simulink model "linear_observor"  (R2023a)
settings: Solver=VariableStepAuto  StartTime=0.0  StopTime=50  RelTol=1e-3
settings Model: Creator=belov  LastModifiedBy=belov

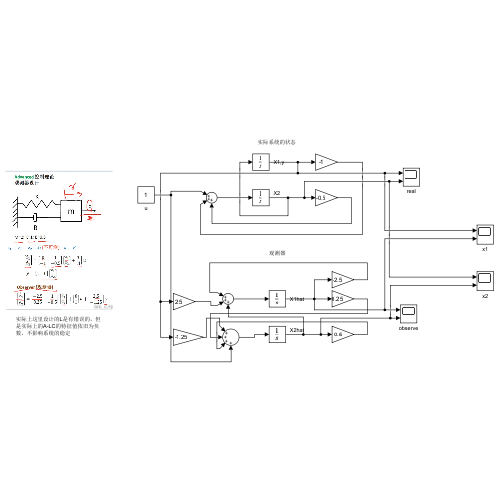
[thumbnail: Simulink's stored preview of the top-level diagram]
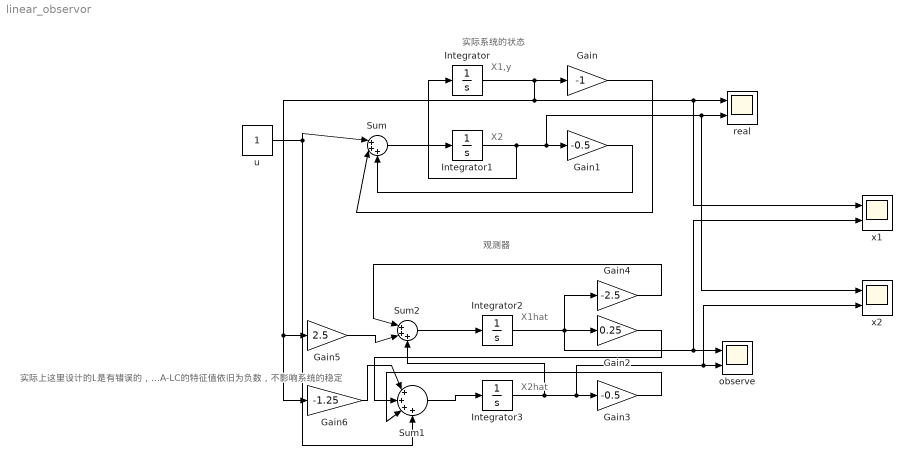
== system linear_observor ==
  note: 实际上这里设计的L是有错误的，但是实际上的A-LC的特征值依旧为负数，不影响系统的稳定
  note: 观测器
  note: 实际系统的状态
  note: X2
  note: X1,y
  note: X2hat
  note: X1hat
  Gain : Gain  Gain=-1
  Gain1 : Gain  Gain=-0.5
  Gain2 : Gain  Gain=0.25
  Gain3 : Gain  Gain=-0.5
  Gain4 : Gain  Gain=-2.5
  Gain5 : Gain  Gain=2.5
  Gain6 : Gain  Gain=-1.25
  Integrator{,1..3} (4 alike) : Integrator
  Sum : Sum  Inputs=|+++
  Sum1 : Sum  Inputs=|++++
  Sum2 : Sum  Inputs=|+++
  observe : Scope  NumInputPorts=2
  real : Scope  NumInputPorts=2
  u : Constant
  x1 : Scope  NumInputPorts=2
  x2 : Scope  NumInputPorts=2
  wires:
  Integrator1/1 -> Integrator/1, x2/1, real/2, Gain1/1
  Integrator/1 -> Gain6/1, Gain5/1, x1/1, real/1, Gain/1
  Sum/1 -> Integrator1/1
  Gain/1 -> Sum/2
  Gain1/1 -> Sum/3
  u/1 -> Sum/1, Sum1/4
  Gain3/1 -> Sum1/3
  Gain2/1 -> Sum1/2
  Sum1/1 -> Integrator3/1
  Integrator3/1 -> Sum2/3, x2/2, observe/2, Gain3/1
  Integrator2/1 -> Gain4/1, x1/2, observe/1, Gain2/1
  Gain4/1 -> Sum2/1
  Sum2/1 -> Integrator2/1
  Gain5/1 -> Sum2/2
  Gain6/1 -> Sum1/1
